simulink model "linear_lung_tube_model"  (R2020a)
settings: Solver=VariableStepAuto  StartTime=0.0  StopTime=finalTime  RelTol=1e-3
values from neighbouring files (symbols this model uses):
  El = 1/50    (= 0.02)    [linear_lung_tube.m]
  Et = 1/2    (= 0.5)    [linear_lung_tube.m]
  Pm_power = 10^-6    (= 1e-06)    [linear_lung_tube.m]
  Q = 200    [linear_lung_tube.m]
  Rl = 2/1000    (= 0.002)    [linear_lung_tube.m]
  Rt = Rl/100    (= 2e-05)    [linear_lung_tube.m]
  T = 4    [linear_lung_tube.m]
libraries: simulink x2
settings Model: Creator=bruno  LastModifiedBy=bruno

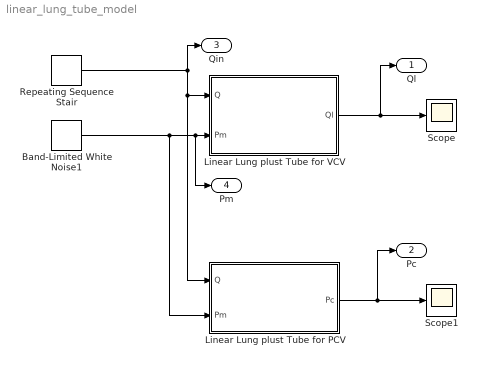
== system linear_lung_tube_model ==
  Band-Limited White Noise1 : simulink/Sources/Band-Limited White Noise  Cov=[Pm_power]  Ts=0.05  seed=[23341]
  Linear Lung plust Tube for PCV : Subsystem
  Linear Lung plust Tube for VCV : Subsystem
  Repeating Sequence Stair : simulink/Sources/Repeating Sequence Stair  OutValues=[Q Q 0 -Q -Q].'  tsamp=T/5  OutMin=[]  OutMax=[]  OutDataTypeStr=double  OutputDataTypeScalingMode=double  OutDataType=fixdt(0,8)  ConRadixGroup=Best Precision: Vector-wise  OutScaling=2^-12
  Scope : Scope
  Scope1 : Scope
  Ql : Outport  SignalName=Ql
  Pc : Outport  Port=2  SignalName=Pc
  Qin : Outport  Port=3  SignalName=Qin
  Pm : Outport  Port=4  SignalName=Pm_in
  wires:
  Linear Lung plust Tube for VCV/1(Ql) -> Ql/1, Scope/1
  Band-Limited White Noise1/1 -> Linear Lung plust Tube for PCV/2(Pm), Pm/1, Linear Lung plust Tube for VCV/2(Pm)
  Linear Lung plust Tube for PCV/1(Pc) -> Pc/1, Scope1/1
  Repeating Sequence Stair/1 -> Linear Lung plust Tube for PCV/1(Q), Linear Lung plust Tube for VCV/1(Q), Qin/1

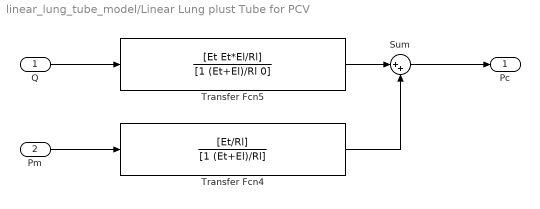
== system linear_lung_tube_model/Linear Lung plust Tube for PCV ==
  Q : Inport
  Pm : Inport  Port=2
  Sum : Sum  Inputs=|++
  Transfer Fcn4 : TransferFcn  Numerator=[Et/Rl]  Denominator=[1 (Et+El)/Rl]
  Transfer Fcn5 : TransferFcn  Numerator=[Et Et*El/Rl]  Denominator=[1 (Et+El)/Rl 0]
  Pc : Outport
  wires:
  Sum/1 -> Pc/1
  Transfer Fcn4/1 -> Sum/2
  Pm/1 -> Transfer Fcn4/1
  Transfer Fcn5/1 -> Sum/1
  Q/1 -> Transfer Fcn5/1

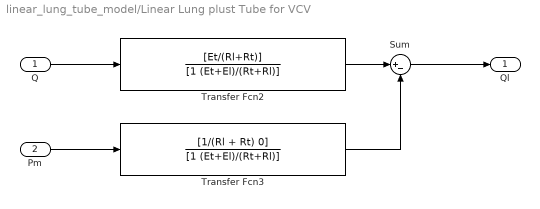
== system linear_lung_tube_model/Linear Lung plust Tube for VCV ==
  Q : Inport
  Pm : Inport  Port=2
  Sum : Sum  Inputs=|+-
  Transfer Fcn2 : TransferFcn  Numerator=[Et/(Rl+Rt)]  Denominator=[1 (Et+El)/(Rt+Rl)]
  Transfer Fcn3 : TransferFcn  Numerator=[1/(Rl + Rt) 0]  Denominator=[1 (Et+El)/(Rt+Rl)]
  Ql : Outport
  wires:
  Sum/1 -> Ql/1
  Transfer Fcn3/1 -> Sum/2
  Pm/1 -> Transfer Fcn3/1
  Transfer Fcn2/1 -> Sum/1
  Q/1 -> Transfer Fcn2/1
